simulink model "q9_2019"  (R2023b)
settings: Solver=VariableStepAuto  StartTime=0.0  StopTime=10.0  RelTol=1e-3
undefined symbols (not defined in the file or in its folder): f1, f2, T
settings Model: Creator=admin  LastModifiedBy=admin

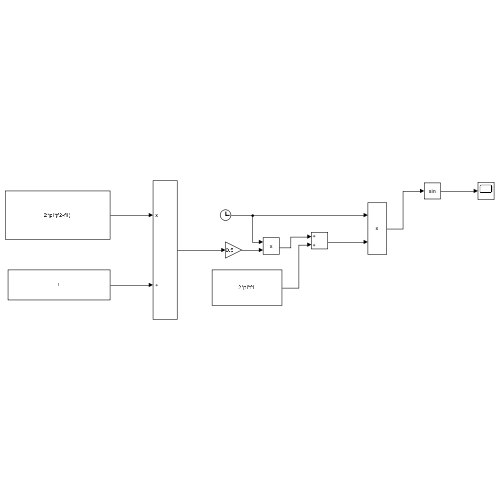
[thumbnail: Simulink's stored preview of the top-level diagram]
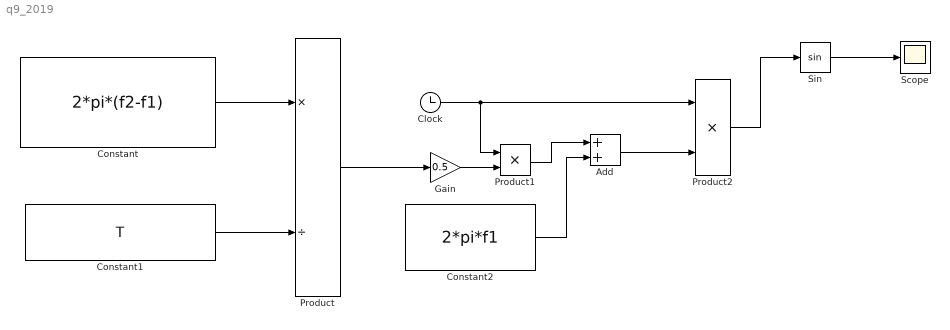
== system q9_2019 ==
  Add : Sum
  Clock : Clock
  Constant : Constant  Value=2*pi*(f2-f1)
  Constant1 : Constant  Value=T
  Constant2 : Constant  Value=2*pi*f1
  Gain : Gain  Gain=0.5
  Product : Product  Inputs=*/
  Product1 : Product
  Product2 : Product
  Scope : Scope
  Sin : Trigonometry
  wires:
  Constant/1 -> Product/1
  Constant1/1 -> Product/2
  Product/1 -> Gain/1
  Gain/1 -> Product1/2
  Clock/1 -> Product1/1, Product2/1
  Product1/1 -> Add/1
  Constant2/1 -> Add/2
  Add/1 -> Product2/2
  Product2/1 -> Sin/1
  Sin/1 -> Scope/1
